simulink model "WiperSystemCtrl"  (R2022b)
settings: Solver=VariableStepAuto  StartTime=0.0  StopTime=10.0  RelTol=1e-3
settings Model: Creator=ahmed  LastModifiedBy=ahmed

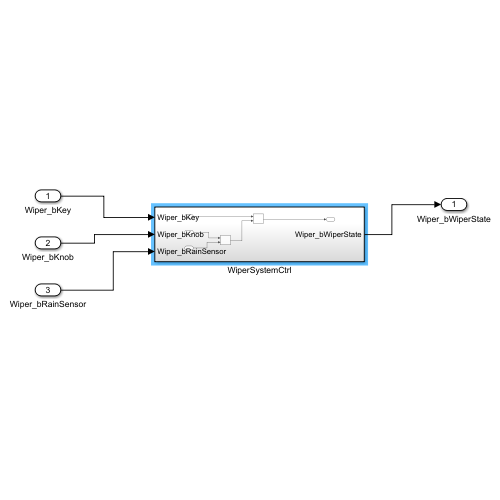
[thumbnail: Simulink's stored preview of the top-level diagram]
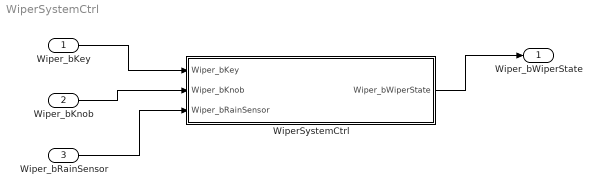
== system WiperSystemCtrl ==
  Wiper_bKey : Inport
  Wiper_bKnob : Inport  Port=2
  Wiper_bRainSensor : Inport  Port=3
  WiperSystemCtrl : Subsystem
  Wiper_bWiperState : Outport
  wires:
  Wiper_bKey/1 -> WiperSystemCtrl/1(Wiper_bKey)
  Wiper_bKnob/1 -> WiperSystemCtrl/2(Wiper_bKnob)
  Wiper_bRainSensor/1 -> WiperSystemCtrl/3(Wiper_bRainSensor)
  WiperSystemCtrl/1(Wiper_bWiperState) -> Wiper_bWiperState/1

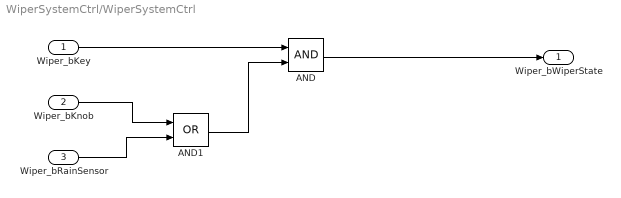
== system WiperSystemCtrl/WiperSystemCtrl ==
  Wiper_bKey : Inport
  Wiper_bKnob : Inport  Port=2
  Wiper_bRainSensor : Inport  Port=3
  AND : Logic  AllPortsSameDT=off  OutDataTypeStr=boolean
  AND1 : Logic  Operator=OR  AllPortsSameDT=off  OutDataTypeStr=boolean
  Wiper_bWiperState : Outport
  wires:
  Wiper_bKnob/1 -> AND1/1
  AND1/1 -> AND/2
  AND/1 -> Wiper_bWiperState/1
  Wiper_bRainSensor/1 -> AND1/2
  Wiper_bKey/1 -> AND/1
